simulink model "sim7"  (R2015b)
settings: Solver=VariableStepAuto  StartTime=0.0  StopTime=T  RelTol=1e-3
values from neighbouring files (symbols this model uses):
  b = 0.025    [Lab2.m]
  dy_inicial = 0    [Lab2.m]
  y_inicial = 1    [Lab2.m]
settings Model: Creator=Alice  LastModifiedBy=Alice

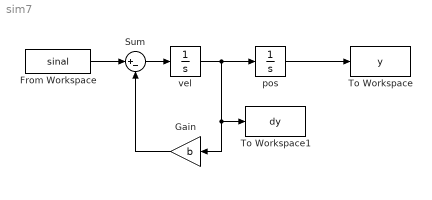
== system sim7 ==
  From Workspace : FromWorkspace  VariableName=sinal  SampleTime=0
  Gain : Gain  Gain=b
  Sum : Sum  Inputs=|+-
  To Workspace : ToWorkspace  VariableName=y  SampleTime=-1
      settings: Save2DSignal=2-D array (concatenate along first dimension)
  To Workspace1 : ToWorkspace  VariableName=dy  SampleTime=-1
      settings: Save2DSignal=2-D array (concatenate along first dimension)
  pos : Integrator  InitialCondition=y_inicial
  vel : Integrator  InitialCondition=dy_inicial
  wires:
  vel/1 -> Gain/1, To Workspace1/1, pos/1
  pos/1 -> To Workspace/1
  Sum/1 -> vel/1
  From Workspace/1 -> Sum/1
  Gain/1 -> Sum/2
